simulink model "Inverter"  (R2016a)
settings: Solver=ode23t  StartTime=0.0  StopTime=1  FixedStep=t_PWM/10  MaxStep=2e-6  RelTol=2e-4
values from neighbouring files (symbols this model uses):
  Rs = sol(3)    [SolarPanelModel.m]
  t_PWM = 20e-6    (= 2e-05)    [SolarPanelModel.m]
undefined symbols (not defined in the file or in its folder): Cdc_inv, Ci, GAMA, k_A, k_inv, Li, Po, Vgrid
libraries: powerlib x7, powerlib_meascontrol x1
settings Model: Creator=frede  LastModifiedBy=frede
settings DataIOCC: LimitDataPoints=on  SaveFormat=Array
settings HardwareCC: ProdBitPerPointer=32  ProdLargestAtomicFloat=None  ProdIntDivRoundTo=Undefined  ProdEndianess=Unspecified  ProdWordSize=32  ProdHWDeviceType=32-bit Generic
settings ModelReferenceCC: PropagateSignalLabelsOutOfModel=off
settings ConfigComp: CovModelRefEnable=Off

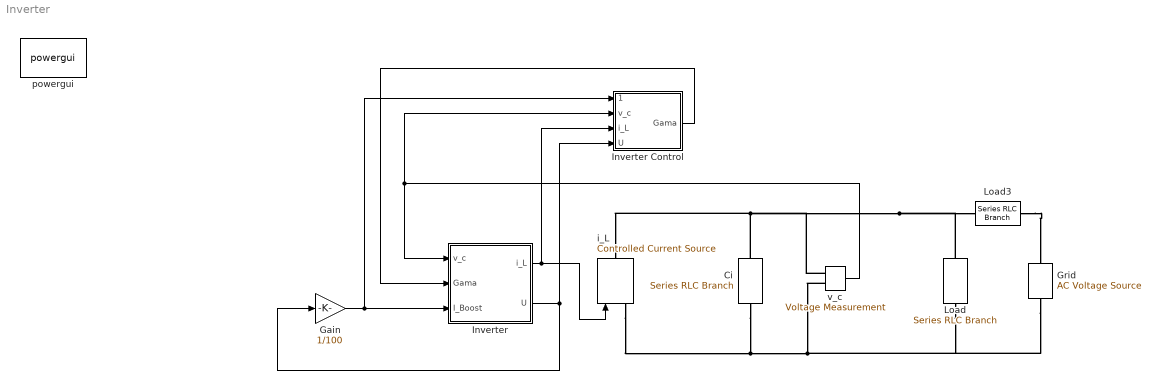
== system Inverter ==
  Ci : powerlib/Elements/Series RLC Branch  LConnTagsString=__new0  RConnTagsString=__new0  BranchType=C  Resistance=Rs  Inductance=1e-3  SetiL0=off  InitialCurrent=0  Capacitance=Ci  Setx0=off  InitialVoltage=0  Measurements=None
  Gain : Gain  Gain=1/100
  Grid : powerlib/Electrical Sources/AC Voltage Source  Amplitude=230*sqrt(2)  Phase=0  Frequency=50  SampleTime=0  Measurements=None  BusType=swing  Pref=10e3  Qref=0  Qmin=-inf  Qmax=+inf
  Inverter : Subsystem
  Inverter Control : Subsystem
  Load : powerlib/Elements/Series RLC Branch  LConnTagsString=__new0  RConnTagsString=__new0  BranchType=R  Resistance=Vgrid^2/Po  Inductance=1e-3  SetiL0=off  InitialCurrent=0  Capacitance=1e-6  Setx0=off  InitialVoltage=0  Measurements=None
  Load3 : powerlib/Elements/Series RLC Branch  LConnTagsString=__new0  RConnTagsString=__new0  BranchType=R  Resistance=0.001  Inductance=1e-3  SetiL0=off  InitialCurrent=0  Capacitance=1e-6  Setx0=off  InitialVoltage=0  Measurements=None
  i_L : powerlib/Electrical Sources/Controlled Current Source  Initialize=on  Source_Type=AC  Amplitude=0  Phase=0  Frequency=0  Measurements=None
  powergui : powerlib/powergui  Priority=1  SimulationMode=Discrete  SolverType=Tustin/Backward Euler (TBE)  SampleTime=t_PWM/10  frequency=60  SPID=off  DisableSnubberDevices=off  DisableRonSwitches=off  DisableVfSwitches=off  SwTol=0  DisplayEquations=off  Interpol=off  ExternalGateDelay=off  methode=off  Ts=10  FunctionMessages=off  echomessages=off  HookPort=off  EnableUseOfTLC=off  x0status=blocks  frequencyindice=0  Pbase=100e6  ErrMax=1e-4  Iterations=50  UnitsV=kV  UnitsW=MW  buscounter=0  RestoreLinks=warning  ResistiveCurrentMeasurement=off  Frange=[0:2:500]  Ylog=off  Xlog=on  ShowGrid=off  save=off  variable=ZData  structure=0  ZoomFFT=off  StartTime=0.0  cycles=1  DisplayStyle=1  fundamental=60  FreqAxis=off  MaxFrequency=1000  frequencyindicesteady=1  RmsSteady=1  display=off
  v_c : powerlib/Measurements/Voltage Measurement  PhasorSimulation=off  OutputType=Complex  PSBequivalent=0
  wires:
  v_c/1 -> Inverter/1(v_c), Inverter Control/2(v_c)
  Inverter/1(i_L) -> i_L/1, Inverter Control/3(i_L)
  Inverter Control/1(Gama) -> Inverter/2(Gama)
  Inverter/2(U) -> Gain/1, Inverter Control/4(U)
  Gain/1 -> Inverter/3(I_Boost), Inverter Control/1(I_boost)
  connections:
  i_L/LConn1 -- Ci/RConn1 -- v_c/LConn2 -- Load/RConn1 -- Grid/LConn1
  Load3/RConn1 -- Grid/RConn1
  Load3/LConn1 -- Load/LConn1 -- v_c/LConn1 -- Ci/LConn1 -- i_L/RConn1

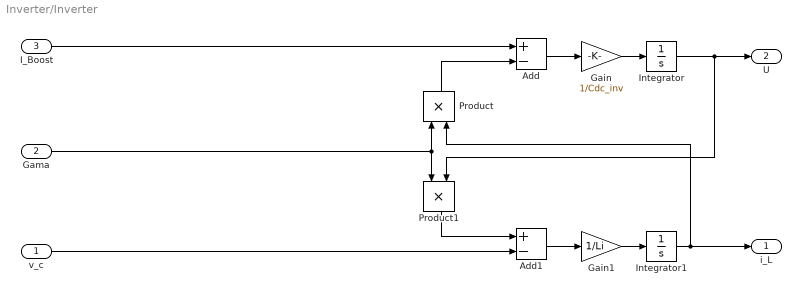
== system Inverter/Inverter ==
  v_c : Inport
  Gama : Inport  Port=2
  I_Boost : Inport  Port=3
  Add : Sum  Inputs=+-
  Add1 : Sum  Inputs=+-
  Gain : Gain  Gain=1/Cdc_inv
  Gain1 : Gain  Gain=1/Li
  Integrator : Integrator  InitialCondition=400  LowerSaturationLimit=0
  Integrator1 : Integrator  LowerSaturationLimit=0
  Product : Product
  Product1 : Product
  i_L : Outport
  U : Outport  Port=2
  wires:
  Integrator1/1 -> i_L/1, Product/2
  Gain/1 -> Integrator/1
  Gain1/1 -> Integrator1/1
  Add/1 -> Gain/1
  Add1/1 -> Gain1/1
  Product/1 -> Add/2
  I_Boost/1 -> Add/1
  Product1/1 -> Add1/1
  v_c/1 -> Add1/2
  Integrator/1 -> Product1/2, U/1
  Gama/1 -> Product1/1, Product/1

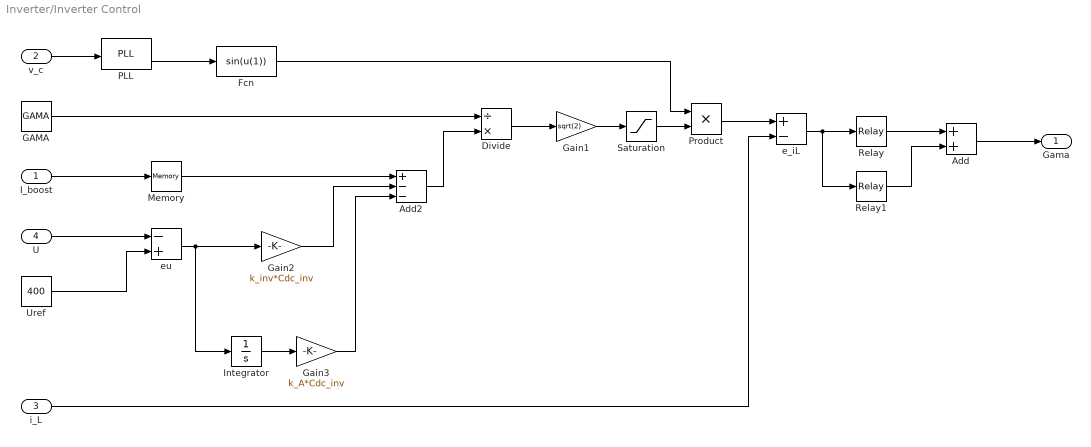
== system Inverter/Inverter Control ==
  I_boost : Inport
  v_c : Inport  Port=2
  i_L : Inport  Port=3
  U : Inport  Port=4
  Add : Sum
  Add2 : Sum  Inputs=+--
  Divide : Product  Inputs=/*
  Fcn : Fcn  Expr=sin(u(1))
  GAMA : Constant  Value=GAMA
  Gain1 : Gain  Gain=sqrt(2)
  Gain2 : Gain  Gain=k_inv*Cdc_inv
  Gain3 : Gain  Gain=k_A*Cdc_inv
  Integrator : Integrator  LimitOutput=on  UpperSaturationLimit=30  LowerSaturationLimit=-30
  Memory : Memory
  PLL : powerlib_meascontrol/PLL/PLL  Fmin=45  Par_Init=[0, 50]  ParK=[180, 3200, 1]  TcD=1e-4  MaxRateChangeFreq=12  FilterCutOffFreq=25  Ts=0  AGC=on
  Product : Product
  Relay : Relay  OnSwitchValue=1.5  OffSwitchValue=-1.5  OnOutputValue=0.5  OffOutputValue=-0.5  ZeroCross=off
  Relay1 : Relay  OnSwitchValue=0.75  OffSwitchValue=-0.75  OnOutputValue=0.5  OffOutputValue=-0.5  ZeroCross=off
  Saturation : Saturate  UpperLimit=30  LowerLimit=-30
  Uref : Constant  Value=400
  e_iL : Sum  Inputs=+-
  eu : Sum  Inputs=-+
  Gama : Outport
  wires:
  e_iL/1 -> Relay1/1, Relay/1
  i_L/1 -> e_iL/2
  Relay/1 -> Add/1
  Relay1/1 -> Add/2
  Add/1 -> Gama/1
  v_c/1 -> PLL/1
  PLL/2 -> Fcn/1
  Product/1 -> e_iL/1
  Fcn/1 -> Product/1
  eu/1 -> Integrator/1, Gain2/1
  Gain2/1 -> Add2/2
  Add2/1 -> Divide/2
  Uref/1 -> eu/2
  GAMA/1 -> Divide/1
  I_boost/1 -> Memory/1
  Divide/1 -> Gain1/1
  Gain1/1 -> Saturation/1
  Memory/1 -> Add2/1
  Saturation/1 -> Product/2
  U/1 -> eu/1
  Integrator/1 -> Gain3/1
  Gain3/1 -> Add2/3
